simulink model "PID_metode_analitik"  (R2021b)
settings: Solver=VariableStepAuto  StartTime=0.0  StopTime=1000  RelTol=1e-3
settings Model: Creator=Asus  LastModifiedBy=Asus

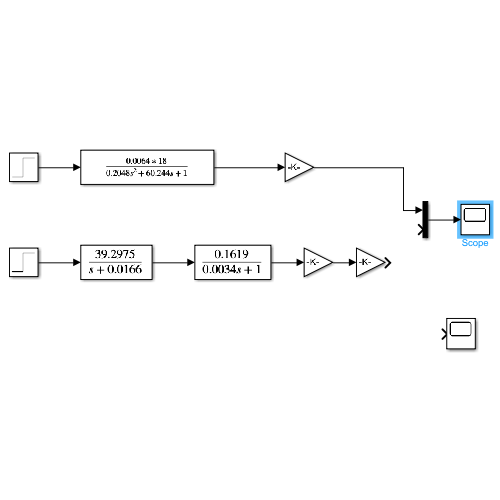
[thumbnail: Simulink's stored preview of the top-level diagram]
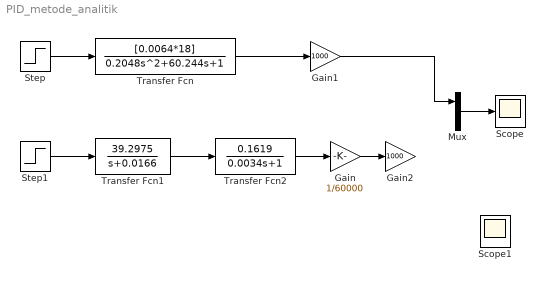
== system PID_metode_analitik ==
  Gain : Gain  Gain=1/60000
  Gain1 : Gain  Gain=1000
  Gain2 : Gain  Gain=1000
  Mux : Mux  Inputs=2
  Scope : Scope
  Scope1 : Scope
  Step : Step  SampleTime=0
  Step1 : Step  After=18  SampleTime=0
  Transfer Fcn : TransferFcn  Numerator=[0.0064*18]  Denominator=[0.2048 60.244 1]
  Transfer Fcn1 : TransferFcn  Numerator=[39.2975]  Denominator=[1 0.0166]
  Transfer Fcn2 : TransferFcn  Numerator=[0.1619]  Denominator=[0.0034 1]
  wires:
  Step/1 -> Transfer Fcn/1
  Transfer Fcn/1 -> Gain1/1
  Transfer Fcn2/1 -> Gain/1
  Transfer Fcn1/1 -> Transfer Fcn2/1
  Step1/1 -> Transfer Fcn1/1
  Mux/1 -> Scope/1
  Gain1/1 -> Mux/1
  Gain/1 -> Gain2/1
